simulink model "APSA"  (R2014b)
settings: Solver=FixedStepDiscrete  StartTime=0.0  StopTime=180  FixedStep=0.01  RelTol=1e-3
PreLoadFcn:
  | if exist('tl_preloadfcn','file'), tl_preloadfcn(gcs,400); end
PostLoadFcn:
  | if exist('tl_postloadfcn','file'), tl_postloadfcn(gcs,400); end
InitFcn:
  | if exist('tlds_init','file'), tlds_init(gcs); end
StartFcn:
  | if exist('tlds_start','file'), tlds_start(gcs); end
StopFcn:
  | if exist('tlds_stop','file'), tlds_stop(gcs); end
values from neighbouring files (symbols this model uses):
  EERAM_Map_Backward_Values = EERAM_Current_Map_Backward.signals.values(row,:)    [Create_Map.m]    (also in EERAM_Map_Backward_Values_2.mat = [0 0 0 0 0 0 150 150 150 150 150 150 ... (100 elements, 1x10)
  EERAM_Map_Forward_Values = EERAM_Current_Map_Forward.signals.values(row,:)    [Create_Map.m]    (also in EERAM_Map_Forward_Values_2.mat = [150 150 150 150 150 150 150 150 150 150 150 150 ... (100 el)
undefined symbols (not defined in the file or in its folder): sigbuilder_block
libraries: tllib x2
(part 1 of 3)
PreSaveFcn:
  | if exist('tl_presavefcn','file'), tl_presavefcn(gcs); end
settings Model: TL_MAIN_DATA={'codeopt',{'linebreaklimit',150,'cleancode',1},'logopt',{'globalloggingmode',4},'date',736348.7418854282,'advcodeopt',{'EnableExternCStateflowSymbols';'on'}}  TLRevision=400  DS_PROJECTFILE=APSA.dd  BufferReuse=off  Creator=VMware  LastModifiedBy=mdenichilo
settings DataIOCC: LimitDataPoints=off
settings OptimizationCC: BlockReduction=off  OptimizeBlockIOStorage=off  BufferReuse=off  GlobalBufferReuse=off  ExpressionFolding=off  LocalBlockOutputs=off
settings DebuggingCC: BusObjectLabelMismatch=error  StrictBusMsg=ErrorOnBusTreatedAsVector  NonBusSignalsTreatedAsBus=error
settings SFSimCC: SimCustomHeaderCode="#include \"APSA_Config.h\""

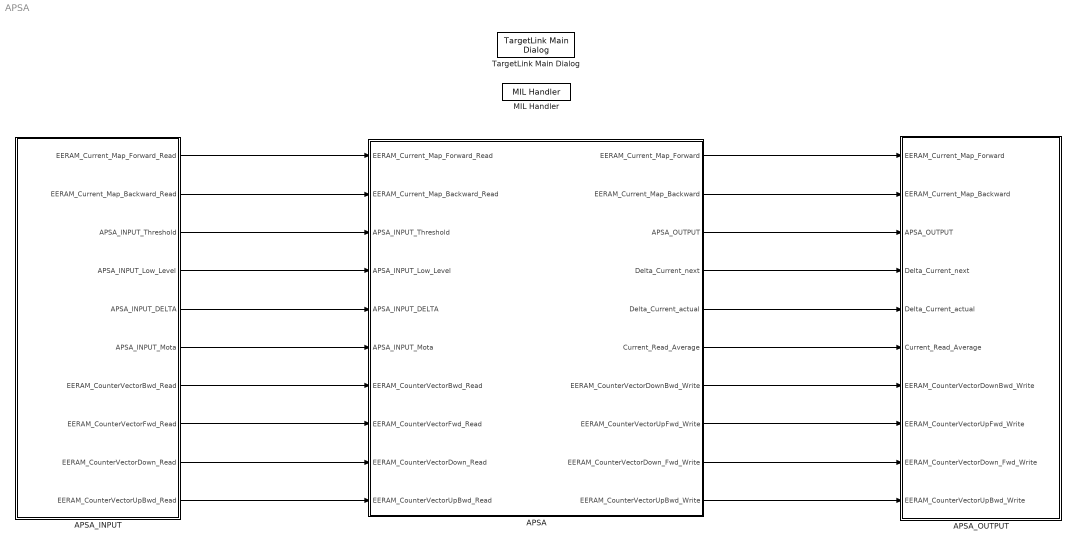
== system APSA ==
  APSA : Subsystem  Tag=TargetLink Simulation Frame  mask(TL_SimFrame){}
      settings: CopyFcn=if exist('tl_copyfcn','file'), tl_copyfcn(gcbh); end  NameChangeFcn=if exist('tl_framenamechangefcn','file'), tl_framenamechangefcn(gcbh); end
      settings: OpenFcn=|
      | if exist('open_tlsubsystem','file')
      |    open_tlsubsystem(gcbh);
      | else
      |    tlsubsystem = ...
      |       find_system(gcb, ...
      |       'LookUnderMasks','on', ...
      |       'FollowLinks','on', ...
      |       'Tag','MIL Subsystem');
      |    open_system(tlsubsystem);
      | end
      mask Display: disp('TargetLink\nModel-\nin-the-loop\nmode')
  APSA_INPUT : Subsystem
  APSA_OUTPUT : Subsystem
  MIL Handler : tllib/MIL Handler  data={'date',730486}
  TargetLink Main Dialog : tllib/TargetLink Main Dialog  data=[]
  wires:
  APSA_INPUT/2(EERAM_Current_Map_Backward_Read) -> APSA/2(EERAM_Current_Map_Backward_Read)
  APSA_INPUT/3(APSA_INPUT_Threshold) -> APSA/3(APSA_INPUT_Threshold)
  APSA_INPUT/6(APSA_INPUT_Mota) -> APSA/6(APSA_INPUT_Mota)
  APSA_INPUT/4(APSA_INPUT_Low_Level) -> APSA/4(APSA_INPUT_Low_Level)
  APSA_INPUT/5(APSA_INPUT_DELTA) -> APSA/5(APSA_INPUT_DELTA)
  APSA_INPUT/1(EERAM_Current_Map_Forward_Read) -> APSA/1(EERAM_Current_Map_Forward_Read)
  APSA/1(EERAM_Current_Map_Forward) -> APSA_OUTPUT/1(EERAM_Current_Map_Forward)
  APSA/2(EERAM_Current_Map_Backward) -> APSA_OUTPUT/2(EERAM_Current_Map_Backward)
  APSA/3(APSA_OUTPUT) -> APSA_OUTPUT/3(APSA_OUTPUT)
  APSA/6(Current_Read_Average) -> APSA_OUTPUT/6(Current_Read_Average)
  APSA/5(Delta_Current_actual) -> APSA_OUTPUT/5(Delta_Current_actual)
  APSA/4(Delta_Current_next) -> APSA_OUTPUT/4(Delta_Current_next)
  APSA/7(EERAM_CounterVectorDownBwd_Write) -> APSA_OUTPUT/7(EERAM_CounterVectorDownBwd_Write)
  APSA/8(EERAM_CounterVectorUpFwd_Write) -> APSA_OUTPUT/8(EERAM_CounterVectorUpFwd_Write)
  APSA/10(EERAM_CounterVectorUpBwd_Write) -> APSA_OUTPUT/10(EERAM_CounterVectorUpBwd_Write)
  APSA/9(EERAM_CounterVectorDown_Fwd_Write) -> APSA_OUTPUT/9(EERAM_CounterVectorDown_Fwd_Write)
  APSA_INPUT/8(EERAM_CounterVectorFwd_Read) -> APSA/8(EERAM_CounterVectorFwd_Read)
  APSA_INPUT/10(EERAM_CounterVectorUpBwd_Read) -> APSA/10(EERAM_CounterVectorUpBwd_Read)
  APSA_INPUT/7(EERAM_CounterVectorBwd_Read) -> APSA/7(EERAM_CounterVectorBwd_Read)
  APSA_INPUT/9(EERAM_CounterVectorDown_Read) -> APSA/9(EERAM_CounterVectorDown_Read)

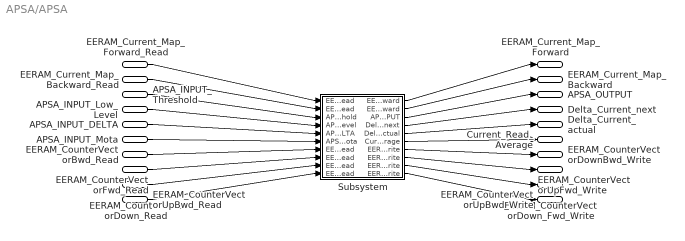
== system APSA/APSA ==
  EERAM_Current_Map_Forward_Read : Inport
  EERAM_Current_Map_Backward_Read : Inport  Port=2
  APSA_INPUT_Threshold : Inport  Port=3
  APSA_INPUT_Low_Level : Inport  Port=4
  APSA_INPUT_DELTA : Inport  Port=5
  APSA_INPUT_Mota : Inport  Port=6
  EERAM_CounterVectorBwd_Read : Inport  Port=7
  EERAM_CounterVectorFwd_Read : Inport  Port=8
  EERAM_CounterVectorDown_Read : Inport  Port=9
  EERAM_CounterVectorUpBwd_Read : Inport  Port=10
  Subsystem : Subsystem  mask(TL_Enable){}
      settings: OpenFcn=warndlg(get_param(gcb,'MaskHelp'),'Serious Warning');
      mask Help: This subsystem keeps the TargetLink subsystem (subsystem with TargetLink blocks for production code generation), and is needed for the TargetLink simulation frame to work properly. DO NOT DELETE OR MODIFY IT!
  EERAM_Current_Map_Forward : Outport
  EERAM_Current_Map_Backward : Outport  Port=2
  APSA_OUTPUT : Outport  Port=3
  Delta_Current_next : Outport  Port=4
  Delta_Current_actual : Outport  Port=5
  Current_Read_Average : Outport  Port=6
  EERAM_CounterVectorDownBwd_Write : Outport  Port=7
  EERAM_CounterVectorUpFwd_Write : Outport  Port=8
  EERAM_CounterVectorDown_Fwd_Write : Outport  Port=9
  EERAM_CounterVectorUpBwd_Write : Outport  Port=10
  wires:
  EERAM_Current_Map_Forward_Read/1 -> Subsystem/1(EERAM_Current_Map_Forward_Read)
  EERAM_Current_Map_Backward_Read/1 -> Subsystem/2(EERAM_Current_Map_Backward_Read)
  APSA_INPUT_Threshold/1 -> Subsystem/3(APSA_INPUT_Threshold)
  APSA_INPUT_Low_Level/1 -> Subsystem/4(APSA_INPUT_Low_Level)
  APSA_INPUT_DELTA/1 -> Subsystem/5(APSA_INPUT_DELTA)
  APSA_INPUT_Mota/1 -> Subsystem/6(APSA_INPUT_Mota)
  EERAM_CounterVectorBwd_Read/1 -> Subsystem/7(EERAM_CounterVectorBwd_Read)
  EERAM_CounterVectorFwd_Read/1 -> Subsystem/8(EERAM_CounterVectorFwd_Read)
  EERAM_CounterVectorDown_Read/1 -> Subsystem/9(EERAM_CounterVectorDown_Read)
  EERAM_CounterVectorUpBwd_Read/1 -> Subsystem/10(EERAM_CounterVectorUpBwd_Read)
  Subsystem/1(EERAM_Current_Map_Forward) -> EERAM_Current_Map_Forward/1
  Subsystem/2(EERAM_Current_Map_Backward) -> EERAM_Current_Map_Backward/1
  Subsystem/3(APSA_OUTPUT) -> APSA_OUTPUT/1
  Subsystem/4(Delta_Current_next) -> Delta_Current_next/1
  Subsystem/5(Delta_Current_actual) -> Delta_Current_actual/1
  Subsystem/6(Current_Read_Average) -> Current_Read_Average/1
  Subsystem/7(EERAM_CounterVectorDownBwd_Write) -> EERAM_CounterVectorDownBwd_Write/1
  Subsystem/8(EERAM_CounterVectorUpFwd_Write) -> EERAM_CounterVectorUpFwd_Write/1
  Subsystem/9(EERAM_CounterVectorDown_Fwd_Write) -> EERAM_CounterVectorDown_Fwd_Write/1
  Subsystem/10(EERAM_CounterVectorUpBwd_Write) -> EERAM_CounterVectorUpBwd_Write/1

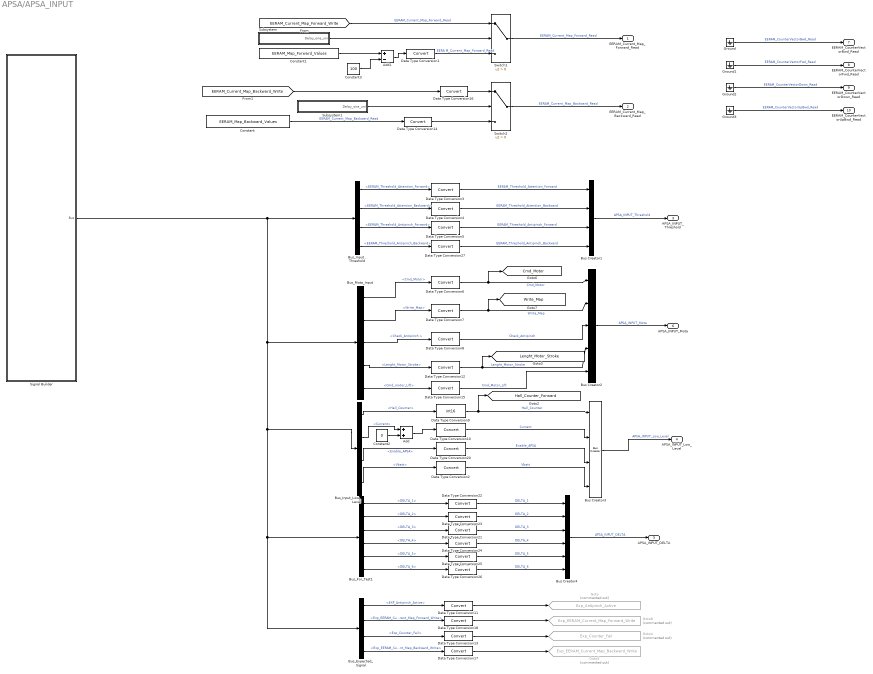
== system APSA/APSA_INPUT ==
  Add : Sum
  Add1 : Sum  Inputs=+-
  Bus Creator1 : BusCreator
  Bus Creator2 : BusCreator  Inputs=5
  Bus Creator3 : BusCreator
  Bus Creator4 : BusCreator  Inputs=6
  Bus_Expected_Signal : BusSelector  OutputSignals=EXP_Antipinch_Active,Exp_EERAM_Current_Map_Forward_Write,Exp_Counter_Fail,Exp_EERAM_Current_Map_Backward_Write
  Bus_For_Test1 : BusSelector  OutputSignals=DELTA_1,DELTA_2,DELTA_3,DELTA_4,DELTA_5,DELTA_6
  Bus_Input_Low_Level : BusSelector  OutputSignals=Hall_Counter,Current,Enable_APSA,Vbatt
  Bus_Input_Threshold : BusSelector  OutputSignals=EERAM_Threshold_Attention_Forward,EERAM_Threshold_Attention_Backward,EERAM_Threshold_Antipinch_Forward,EERAM_Threshold_Antipinch_Backward
  Bus_Mota_Input : BusSelector  OutputSignals=Cmd_Motor,Write_Map,Check_Antipinch ,Lenght_Motor_Stroke,Cmd_motor_Lift
  Constant : Constant  Value=EERAM_Map_Backward_Values  OutDataTypeStr=double
  Constant1 : Constant  Value=EERAM_Map_Forward_Values  OutDataTypeStr=double
  Constant2 : Constant  Value=0
  Constant3 : Constant  Value=100
  Data Type Conversion{1..8,10..18,20..27} (25 alike) : DataTypeConversion
  Data Type Conversion9 : DataTypeConversion  OutDataTypeStr=int16
  Goto : Goto  Commented=on  GotoTag=Exp_Antipinch_Active  TagVisibility=global
  Goto4 : Goto  Commented=on  GotoTag=Exp_Counter_Fail  TagVisibility=global
  Goto5 : Goto  Commented=on  GotoTag=Exp_EERAM_Current_Map_Backward_Write  TagVisibility=global
  Goto8 : Goto  Commented=on  GotoTag=Exp_EERAM_Current_Map_Forward_Write  TagVisibility=global
  Ground{,1..3} (4 alike) : Ground
  Signal Builder : Subsystem  Tag=STV Subsys  LoadFcn=sigbuilder_block('load');  StartFcn=sigbuilder_block('start');  StopFcn=sigbuilder_block('stop');  ClipboardFcn=sigbuilder_block('clipboard');  mask(Sigbuilder block){}
      mask help: Simulink:masks:SigbuilderBlock_MD
      mask init:
      | if ~strcmp(get_param(bdroot(gcbh),'SimulationStatus'),'stopped') tuvar = sigbuilder_block('maskInit'); end
      settings: CopyFcn=sigbuilder_block('copy');  DeleteFcn=sigbuilder_block('delete');  ModelCloseFcn=sigbuilder_block('modelClose');  PreSaveFcn=sigbuilder_block('preSave');  PauseFcn=sigbuilder_block('pause');  ContinueFcn=sigbuilder_block('continue');  NameChangeFcn=sigbuilder_block('namechange');  OpenFcn=sigbuilder_block('open',[437.6 199.2 550.4 400 ]);  CloseFcn=sigbuilder_block('close');
      mask Display: plot(0, 0, 100, 100,[2, 2, 32, 32, 2], [68, 8, 8, 68, 68],[32, 2], [38, 38], [32, 19, 2],[53, 60, 44], [32, 17, 17, 2],[16, 16, 31, 31]);txt = getActiveGroup(gcbh);text(2, 100, txt,'verticalAlignment', 'top');
  Subsystem : Subsystem
  Subsystem1 : Subsystem
  Switch1 : Switch  Criteria=u2 > Threshold
  Switch2 : Switch  Criteria=u2 > Threshold
  EERAM_Current_Map_Forward_Read : Outport
  EERAM_Current_Map_Backward_Read : Outport  Port=2
  APSA_INPUT_Threshold : Outport  Port=3
  APSA_INPUT_Low_Level : Outport  Port=4
  APSA_INPUT_DELTA : Outport  Port=5
  APSA_INPUT_Mota : Outport  Port=6
  EERAM_CounterVectorBwd_Read : Outport  Port=7
  EERAM_CounterVectorFwd_Read : Outport  Port=8
  EERAM_CounterVectorDown_Read : Outport  Port=9
  EERAM_CounterVectorUpBwd_Read : Outport  Port=10
  tag scope: Cmd_Motor=global, Hall_Counter_Forward=global, Lenght_Motor_Stroke=global, Write_Map=global
  wires:
  Bus_Input_Threshold/1 -> Data Type Conversion3/1  "<EERAM_Threshold_Attention_Forward>"
  Bus_Input_Threshold/3 -> Data Type Conversion5/1  "<EERAM_Threshold_Antipinch_Forward>"
  Bus_Mota_Input/1 -> Data Type Conversion6/1  "<Cmd_Motor>"
  Bus_Mota_Input/2 -> Data Type Conversion7/1  "<Write_Map>"
  Bus_Mota_Input/3 -> Data Type Conversion8/1  "<Check_Antipinch >"
  Data Type Conversion3/1 -> Bus Creator1/1  "EERAM_Threshold_Attention_Forward"
  Data Type Conversion5/1 -> Bus Creator1/3  "EERAM_Threshold_Antipinch_Forward"
  Data Type Conversion7/1 -> [Write_Map], Bus Creator2/2  "Write_Map"
  Data Type Conversion8/1 -> Bus Creator2/3  "Check_Antipinch"
  Data Type Conversion6/1 -> [Cmd_Motor], Bus Creator2/1  "Cmd_Motor"
  Bus Creator1/1 -> APSA_INPUT_Threshold/1  "APSA_INPUT_Threshold"
  Bus Creator2/1 -> APSA_INPUT_Mota/1  "APSA_INPUT_Mota"
  Bus_Input_Low_Level/1 -> Data Type Conversion9/1  "<Hall_Counter>"
  Bus_Input_Low_Level/2 -> Add/1  "<Current>"
  Data Type Conversion10/1 -> Bus Creator3/2  "Current"
  Data Type Conversion9/1 -> [Hall_Counter_Forward], Bus Creator3/1  "Hall_Counter"
  Bus_Mota_Input/4 -> Data Type Conversion12/1  "<Lenght_Motor_Stroke>"
  Data Type Conversion12/1 -> [Lenght_Motor_Stroke], Bus Creator2/4  "Lenght_Motor_Stroke"
  Bus Creator3/1 -> APSA_INPUT_Low_Level/1  "APSA_INPUT_Low_Level"
  Bus_Expected_Signal/1 -> Data Type Conversion11/1  "<EXP_Antipinch_Active>"
  Data Type Conversion11/1 -> Goto/1
  Bus_Expected_Signal/2 -> Data Type Conversion18/1  "<Exp_EERAM_Current_Map_Forward_Write>"
  Bus_Input_Threshold/2 -> Data Type Conversion4/1  "<EERAM_Threshold_Attention_Backward>"
  Data Type Conversion4/1 -> Bus Creator1/2  "EERAM_Threshold_Attention_Backward"
  Bus_Expected_Signal/3 -> Data Type Conversion13/1  "<Exp_Counter_Fail>"
  Data Type Conversion13/1 -> Goto4/1
  Data Type Conversion1/1 -> Switch1/3  "EERA M_Current_Map_Forward_Read"
  Subsystem/1(Delay_one_unit) -> Switch1/2
  [EERAM_Current_Map_Forward_Write] -> Switch1/1  "EERAM_Current_Map_Forward_Read"
  Signal Builder/1(Bus) -> Bus_Input_Threshold/1, Bus_Input_Low_Level/1, Bus_For_Test1/1, Bus_Expected_Signal/1, Bus_Mota_Input/1
  Subsystem1/1(Delay_one_unit) -> Switch2/2
  [EERAM_Current_Map_Backward_Write] -> Data Type Conversion16/1
  Data Type Conversion16/1 -> Switch2/1
  Bus_Expected_Signal/4 -> Data Type Conversion17/1  "<Exp_EERAM_Current_Map_Backward_Write>"
  Data Type Conversion17/1 -> Goto5/1
  Bus_Input_Low_Level/3 -> Data Type Conversion20/1  "<Enable_APSA>"
  Data Type Conversion20/1 -> Bus Creator3/3  "Enable_APSA"
  Bus_For_Test1/1 -> Data Type Conversion22/1  "<DELTA_1>"
  Bus_For_Test1/2 -> Data Type Conversion23/1  "<DELTA_2>"
  Bus_For_Test1/3 -> Data Type Conversion21/1  "<DELTA_3>"
  Bus_For_Test1/4 -> Data Type Conversion24/1  "<DELTA_4>"
  Bus_For_Test1/5 -> Data Type Conversion25/1  "<DELTA_5>"
  Bus_For_Test1/6 -> Data Type Conversion26/1  "<DELTA_6>"
  Data Type Conversion23/1 -> Bus Creator4/2  "DELTA_2"
  Data Type Conversion26/1 -> Bus Creator4/6  "DELTA_6"
  Data Type Conversion22/1 -> Bus Creator4/1  "DELTA_1"
  Data Type Conversion24/1 -> Bus Creator4/4  "DELTA_4"
  Data Type Conversion25/1 -> Bus Creator4/5  "DELTA_5"
  Data Type Conversion21/1 -> Bus Creator4/3  "DELTA_3"
  Bus Creator4/1 -> APSA_INPUT_DELTA/1  "APSA_INPUT_DELTA"
  Constant1/1 -> Add1/1
  Bus_Input_Threshold/4 -> Data Type Conversion27/1  "<EERAM_Threshold_Antipinch_Backward>"
  Data Type Conversion27/1 -> Bus Creator1/4  "EERAM_Threshold_Antipinch_Backward"
  Constant/1 -> Data Type Conversion14/1  "EERAM_Current_Map_Backward_Read"
  Data Type Conversion18/1 -> Goto8/1
  Switch1/1 -> EERAM_Current_Map_Forward_Read/1  "EERAM_Current_Map_Forward_Read"
  Switch2/1 -> EERAM_Current_Map_Backward_Read/1  "EERAM_Current_Map_Backward_Read"
  Constant2/1 -> Add/2
  Add/1 -> Data Type Conversion10/1
  Constant3/1 -> Add1/2
  Data Type Conversion14/1 -> Switch2/3
  Add1/1 -> Data Type Conversion1/1
  Ground/1 -> EERAM_CounterVectorBwd_Read/1  "EERAM_CounterVectorBwd_Read"
  Ground1/1 -> EERAM_CounterVectorFwd_Read/1  "EERAM_CounterVectorFwd_Read"
  Ground2/1 -> EERAM_CounterVectorDown_Read/1  "EERAM_CounterVectorDown_Read"
  Ground3/1 -> EERAM_CounterVectorUpBwd_Read/1  "EERAM_CounterVectorUpBwd_Read"
  Bus_Input_Low_Level/4 -> Data Type Conversion2/1  "<Vbatt>"
  Data Type Conversion2/1 -> Bus Creator3/4  "Vbatt"
  Bus_Mota_Input/5 -> Data Type Conversion15/1  "<Cmd_motor_Lift>"
  Data Type Conversion15/1 -> Bus Creator2/5  "Cmd_Motor_Lift"

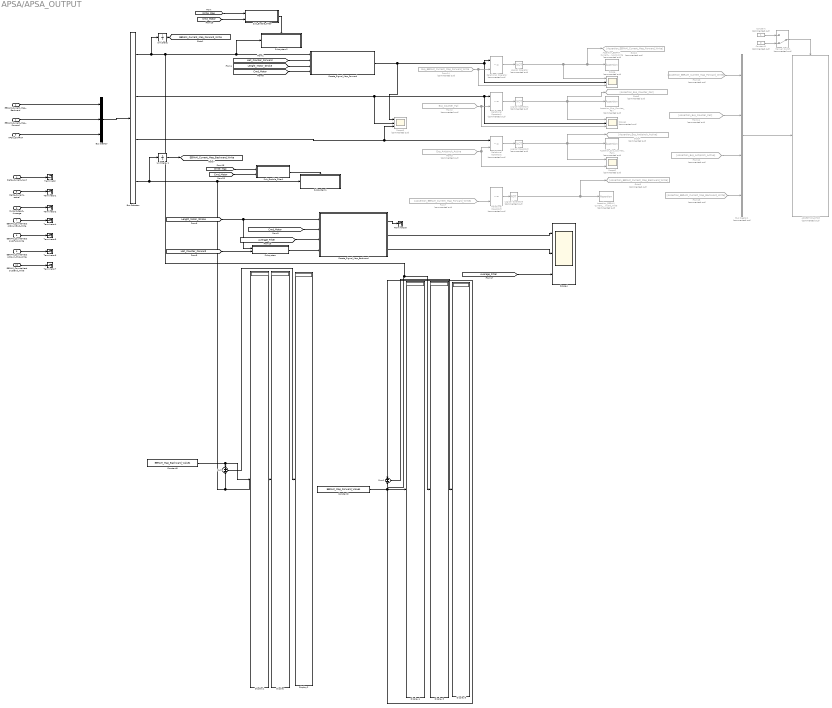
== system APSA/APSA_OUTPUT ==
  EERAM_Current_Map_Forward : Inport
  EERAM_Current_Map_Backward : Inport  Port=2
  APSA_OUTPUT : Inport  Port=3
  Delta_Current_next : Inport  Port=4
  Delta_Current_actual : Inport  Port=5
  Current_Read_Average : Inport  Port=6
  EERAM_CounterVectorDownBwd_Write : Inport  Port=7
  EERAM_CounterVectorUpFwd_Write : Inport  Port=8
  EERAM_CounterVectorDown_Fwd_Write : Inport  Port=9
  EERAM_CounterVectorUpBwd_Write : Inport  Port=10
  ASSERTION_STOP : Subsystem  Commented=on
  Assertion_EERAM_Current_Map_Backward_Write : Assertion  Commented=on  StopWhenAssertionFail=off
  Assertion_EERAM_Current_Map_Forward_Write : Assertion  Commented=on  StopWhenAssertionFail=off
  Assertion_Exp_Counter_Fail : Assertion  Commented=on  StopWhenAssertionFail=off
  Assertion_Exp_Counter_Fail1 : Assertion  Commented=on  StopWhenAssertionFail=off
  Bus Creator : BusCreator  Inputs=3
  Bus Creator1 : BusCreator  Commented=on
  Bus Selector : BusSelector  OutputSignals=EERAM_Current_Map_Forward_Write,APSA_OUTPUT.Fail_Sens_Current,APSA_OUTPUT.Antipinch_Active,EERAM_Current_Map_Backward_Write
  Constant : Constant  Commented=on
  Constant1 : Constant  Commented=on  Value=0
  Constant2 : Constant  Value=EERAM_Map_Forward_Values  OutDataTypeStr=double
  Constant3 : Constant  Value=EERAM_Map_Backward_Values  OutDataTypeStr=double
  Create_Signal_Map_Backward : Stateflow chart  TreatAsAtomicUnit=on
  Create_Signal_Map_Forward : Stateflow chart  TreatAsAtomicUnit=on
  Display{,1..5} (6 alike) : Display
  From10 : From  Commented=on  GotoTag=Assertion_EERAM_Current_Map_Forward_Write
  From11 : From  Commented=on  GotoTag=Assertion_Exp_Counter_Fail
  From12 : From  Commented=on  GotoTag=Assertion_Exp_Antipinch_Active
  From13 : From  Commented=on  GotoTag=Assertion_EERAM_Current_Map_Backward_Write
  From14 : From  Commented=on  GotoTag=Exp_EERAM_Current_Map_Forward_Write
  From2 : From  Commented=on  GotoTag=Exp_Counter_Fail  TagVisibility=global
  From3 : From  Commented=on  GotoTag=Exp_Antipinch_Active  TagVisibility=global
  From7 : From  Commented=on  GotoTag=Assertion_EERAM_Current_Map_Forward_Write
  Goto2 : Goto  Commented=on  GotoTag=Assertion_EERAM_Current_Map_Forward_Write
  Goto3 : Goto  Commented=on  GotoTag=Assertion_Exp_Counter_Fail
  Goto4 : Goto  Commented=on  GotoTag=Assertion_Exp_Antipinch_Active
  Goto5 : Goto  Commented=on  GotoTag=Assertion_EERAM_Current_Map_Backward_Write
  Logical Operator{,1..3} (4 alike) : Logic  Commented=on  Operator=NOT  AllPortsSameDT=off  OutDataTypeStr=boolean
  Manual Switch : ManualSwitch  Commented=on  CurrentSetting=0
  Relational Operator{,1..3} (4 alike) : RelationalOperator  Commented=on  Operator=~=  OutDataTypeStr=boolean
  Scope{,1..3} (4 alike) : Scope  Commented=on  NumInputPorts=3
      Scope settings: TimeRange=0.008849178119752832  YMin=-1~0~5.6  YMax=1~5~5.74  SampleInput=on
      Scope1 settings: YMin=-5~-5~-5  YMax=5~5~5
      Scope2 settings: YMin=-5~-5~-5  YMax=5~5~5  SaveName=ScopeData2
      Scope3 settings: YMin=-5~-5~-5  YMax=5~5~5  SaveName=ScopeData3
  Scope4 : Scope  NumInputPorts=3
      settings: TimeRange=0.1993998881147334  YMin=-1~-1~43  YMax=1~1~47  SaveName=ScopeData5  SampleInput=on
  Sub_Enable_Filter : Subsystem
  Sub_Enable_Filter1 : Subsystem
  Subsystem : Subsystem
  Subsystem1 : Subsystem
  Subsystem2 : Subsystem
  Sum : Sum  Inputs=+-
  Sum1 : Sum  Inputs=+-
  Terminator{,1..7} (8 alike) : Terminator
  Unit Delay : UnitDelay  SampleTime=-1
  Unit Delay1 : UnitDelay  SampleTime=-1
  tag scope: EERAM_Current_Map_Backward_Write=global, EERAM_Current_Map_Forward_Write=global
  wires:
  Logical Operator/1 -> Goto2/1, Assertion_EERAM_Current_Map_Forward_Write/1, Scope/1  "Assertion_EERAM_Current_Map_Forward_Write"
  Relational Operator/1 -> Logical Operator/1
  Create_Signal_Map_Forward/1(Map_Signal) -> Scope3/1, Relational Operator/1, Scope/2
  [Hall_Counter_Forward] -> Create_Signal_Map_Forward/2(Hall_Counter)
  [Lenght_Motor_Stroke] -> Create_Signal_Map_Forward/3(Lenght_Motor_Stroke)
  APSA_OUTPUT/1 -> Bus Creator/3
  Bus Selector/2 -> Scope3/2, Scope1/2, Relational Operator1/1  "<Fail_Sens_Current>"
  From2/1 -> Scope1/3, Relational Operator1/2  "Exp_Counter_Fail"
  Relational Operator1/1 -> Logical Operator1/1
  Logical Operator1/1 -> Scope1/1, Goto3/1, Assertion_Exp_Counter_Fail/1  "Assertion_Exp_Counter_Fail"
  From3/1 -> Scope2/3, Relational Operator2/2  "Exp_Antipinch_Active"
  Relational Operator2/1 -> Logical Operator2/1
  Logical Operator2/1 -> Goto4/1, Scope2/1, Assertion_Exp_Counter_Fail1/1  "Assertion_Exp_Antipinch_Active"
  Bus Selector/4 -> Unit Delay1/1, Display/1, Sum/2, Subsystem1/1(In1)  "<EERAM_Current_Map_Backward_Write>"
  Subsystem/1(Hall_Counter_Backward) -> Create_Signal_Map_Backward/4(Hall_Counter_Backward)
  Logical Operator3/1 -> Goto5/1, Assertion_EERAM_Current_Map_Backward_Write/1  "Assertion_EERAM_Current_Map_Backward_Write"
  Relational Operator3/1 -> Logical Operator3/1
  [Cmd_Motor] -> Create_Signal_Map_Forward/4(Cmd_Motor)
  [Cmd_Motor] -> Create_Signal_Map_Backward/2(Cmd_Motor)
  EERAM_Current_Map_Forward/1 -> Bus Creator/2
  EERAM_Current_Map_Backward/1 -> Bus Creator/1
  Bus Creator/1 -> Bus Selector/1
  [Hall_Counter_Forward] -> Subsystem/2(Hall_Counter)
  Bus Creator1/1 -> ASSERTION_STOP/1(Assertion_Stop)
  From10/1 -> Bus Creator1/1
  From11/1 -> Bus Creator1/2
  From12/1 -> Bus Creator1/3
  From13/1 -> Bus Creator1/4
  Manual Switch/1 -> ASSERTION_STOP/Enable
  Constant/1 -> Manual Switch/1
  Constant1/1 -> Manual Switch/2
  Bus Selector/3 -> Scope3/3, Relational Operator2/1  "<Antipinch_Active>"
  From14/1 -> Scope/3, Relational Operator/2
  From7/1 -> Relational Operator3/2
  [Average_Filter] -> Create_Signal_Map_Backward/3(Current)
  Create_Signal_Map_Backward/2(Index_vector) -> Scope4/1  "indexvector"
  [Average_Filter] -> Scope4/3
  [Lenght_Motor_Stroke] -> Subsystem/1(Lenght_Motor_Stroke), Create_Signal_Map_Backward/1(Lenght_Motor_Stroke)
  Create_Signal_Map_Backward/3(Mappa) -> Scope4/2  "mappa_attuale"
  Sub_Enable_Filter1/1(Enable_Filter) -> Subsystem1/Enable
  Bus Selector/1 -> Unit Delay/1, Sum1/2, Display3/1, Subsystem2/1(In1), Create_Signal_Map_Forward/1(EERAM_Current_Map_Forward_Write)  "<EERAM_Current_Map_Forward_Write>"
  [Write_Map] -> Sub_Enable_Filter/1(Write_Map)
  [Cmd_Motor] -> Sub_Enable_Filter/2(Cmd_Motor)
  Sub_Enable_Filter/1(Enable_Filter) -> Subsystem2/Enable
  [Write_Map] -> Sub_Enable_Filter1/1(Write_Map)
  [Cmd_Motor] -> Sub_Enable_Filter1/2(Cmd_Motor)
  Constant3/1 -> Display1/1, Sum/1
  Delta_Current_next/1 -> Terminator/1
  Delta_Current_actual/1 -> Terminator1/1
  Current_Read_Average/1 -> Terminator2/1
  Sum/1 -> Display2/1
  Constant2/1 -> Sum1/1, Display4/1
  Sum1/1 -> Display5/1
  Create_Signal_Map_Backward/1(EERAM_Current_Map_Backward_Write) -> Terminator3/1
  Unit Delay/1 -> [EERAM_Current_Map_Forward_Write]
  Unit Delay1/1 -> [EERAM_Current_Map_Backward_Write]
  EERAM_CounterVectorDownBwd_Write/1 -> Terminator4/1
  EERAM_CounterVectorUpFwd_Write/1 -> Terminator5/1
  EERAM_CounterVectorDown_Fwd_Write/1 -> Terminator6/1
  EERAM_CounterVectorUpBwd_Write/1 -> Terminator7/1

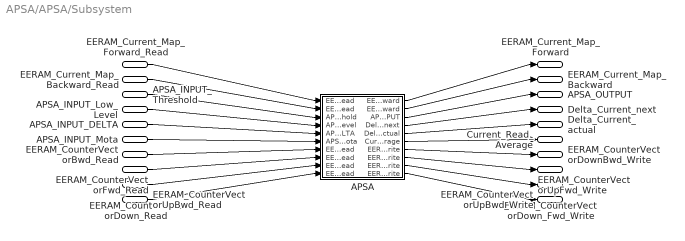
== system APSA/APSA/Subsystem ==
  EERAM_Current_Map_Forward_Read : Inport
  EERAM_Current_Map_Backward_Read : Inport  Port=2
  APSA_INPUT_Threshold : Inport  Port=3
  APSA_INPUT_Low_Level : Inport  Port=4
  APSA_INPUT_DELTA : Inport  Port=5
  APSA_INPUT_Mota : Inport  Port=6
  EERAM_CounterVectorBwd_Read : Inport  Port=7
  EERAM_CounterVectorFwd_Read : Inport  Port=8
  EERAM_CounterVectorDown_Read : Inport  Port=9
  EERAM_CounterVectorUpBwd_Read : Inport  Port=10
  APSA : Subsystem  Tag=MIL Subsystem  Description=a  mask(MIL Subsystem){}
      settings: CopyFcn=if exist('tl_copyfcn','file'), tl_copyfcn(gcbh); end  NameChangeFcn=if exist('tl_namechangefcn','file'), tl_namechangefcn(gcbh); end  DestroyFcn=if exist('update_tl_main_dlg','file'), update_tl_main_dlg('TL_subs_display'); end
      mask Display: disp('TargetLink Subsystem')
  EERAM_Current_Map_Forward : Outport
  EERAM_Current_Map_Backward : Outport  Port=2
  APSA_OUTPUT : Outport  Port=3
  Delta_Current_next : Outport  Port=4
  Delta_Current_actual : Outport  Port=5
  Current_Read_Average : Outport  Port=6
  EERAM_CounterVectorDownBwd_Write : Outport  Port=7
  EERAM_CounterVectorUpFwd_Write : Outport  Port=8
  EERAM_CounterVectorDown_Fwd_Write : Outport  Port=9
  EERAM_CounterVectorUpBwd_Write : Outport  Port=10
  wires:
  EERAM_Current_Map_Forward_Read/1 -> APSA/1(EERAM_Current_Map_Forward_Read)
  EERAM_Current_Map_Backward_Read/1 -> APSA/2(EERAM_Current_Map_Backward_Read)
  APSA_INPUT_Threshold/1 -> APSA/3(APSA_INPUT_Threshold)
  APSA_INPUT_Low_Level/1 -> APSA/4(APSA_INPUT_Low_Level)
  APSA_INPUT_DELTA/1 -> APSA/5(APSA_INPUT_DELTA)
  APSA_INPUT_Mota/1 -> APSA/6(APSA_INPUT_Mota)
  EERAM_CounterVectorBwd_Read/1 -> APSA/7(EERAM_CounterVectorBwd_Read)
  EERAM_CounterVectorFwd_Read/1 -> APSA/8(EERAM_CounterVectorFwd_Read)
  EERAM_CounterVectorDown_Read/1 -> APSA/9(EERAM_CounterVectorDown_Read)
  EERAM_CounterVectorUpBwd_Read/1 -> APSA/10(EERAM_CounterVectorUpBwd_Read)
  APSA/1(EERAM_Current_Map_Forward) -> EERAM_Current_Map_Forward/1
  APSA/2(EERAM_Current_Map_Backward) -> EERAM_Current_Map_Backward/1
  APSA/3(APSA_OUTPUT) -> APSA_OUTPUT/1
  APSA/4(Delta_Current_next) -> Delta_Current_next/1
  APSA/5(Delta_Current_actual) -> Delta_Current_actual/1
  APSA/6(Current_Read_Average) -> Current_Read_Average/1
  APSA/7(EERAM_CounterVectorDownBwd_Write) -> EERAM_CounterVectorDownBwd_Write/1
  APSA/8(EERAM_CounterVectorUpFwd_Write) -> EERAM_CounterVectorUpFwd_Write/1
  APSA/9(EERAM_CounterVectorDown_Fwd_Write) -> EERAM_CounterVectorDown_Fwd_Write/1
  APSA/10(EERAM_CounterVectorUpBwd_Write) -> EERAM_CounterVectorUpBwd_Write/1

== system APSA/APSA_INPUT/Signal Builder ==
  Bus Creator : BusCreator  Tag=Bus Creator  Inputs=28
  FromWs : FromWorkspace  Tag=STV FromWs  VariableName=tuvar  SampleTime=0
  Subsystem : Subsystem
  Bus : Outport
  wires:
  FromWs/1 -> Subsystem/1(In1)
  Bus Creator/1 -> Bus/1
  Subsystem/1(Enable_APSA) -> Bus Creator/1  "Enable_APSA"
  Subsystem/2(Cmd_Motor) -> Bus Creator/2  "Cmd_Motor"
  Subsystem/3(Hall_Counter) -> Bus Creator/3  "Hall_Counter"
  Subsystem/4("Check_Antipinch ") -> Bus Creator/4  "Check_Antipinch"
  Subsystem/5(Current) -> Bus Creator/5  "Current"
  Subsystem/6(Write_Map) -> Bus Creator/6  "Write_Map"
  Subsystem/7(Lenght_Motor_Stroke) -> Bus Creator/7  "Lenght_Motor_Stroke"
  Subsystem/8(EERAM_Threshold_Attention_Forward) -> Bus Creator/8  "EERAM_Threshold_Attention_Forward"
  Subsystem/9(EERAM_Threshold_Attention_Backward) -> Bus Creator/9  "EERAM_Threshold_Attention_Backward"
  Subsystem/10(EERAM_Threshold_Antipinch_Forward) -> Bus Creator/10  "EERAM_Threshold_Antipinch_Forward"
  Subsystem/11(EERAM_Threshold_Antipinch_Backward) -> Bus Creator/11  "EERAM_Threshold_Antipinch_Backward"
  Subsystem/12(DELTA_1) -> Bus Creator/12  "DELTA_1"
  Subsystem/13(DELTA_2) -> Bus Creator/13  "DELTA_2"
  Subsystem/14(DELTA_3) -> Bus Creator/14  "DELTA_3"
  Subsystem/15(Current1) -> Bus Creator/15  "Current1"
  Subsystem/16(DELTA_4) -> Bus Creator/16  "DELTA_4"
  Subsystem/17(DELTA_5) -> Bus Creator/17  "DELTA_5"
  Subsystem/18(DELTA_6) -> Bus Creator/18  "DELTA_6"
  Subsystem/19(EXP_Antipinch_Active) -> Bus Creator/19  "EXP_Antipinch_Active"
  Subsystem/20(Exp_EERAM_Current_Map_Forward_Write) -> Bus Creator/20  "Exp_EERAM_Current_Map_Forward_Write"
  Subsystem/21(Exp_EERAM_Current_Map_Backward_Write) -> Bus Creator/21  "Exp_EERAM_Current_Map_Backward_Write"
  Subsystem/22(Exp_Counter_Fail) -> Bus Creator/22  "Exp_Counter_Fail"
  Subsystem/23(mappa) -> Bus Creator/23  "mappa"
  Subsystem/24(3EEP_10V) -> Bus Creator/24  "3EEP_10V"
  Subsystem/25(3EEP_12V) -> Bus Creator/25  "3EEP_12V"
  Subsystem/26(3xEEP_16V) -> Bus Creator/26  "3xEEP_16V"
  Subsystem/27(Vbatt) -> Bus Creator/27  "Vbatt"
  Subsystem/28(Cmd_motor_Lift) -> Bus Creator/28  "Cmd_motor_Lift"

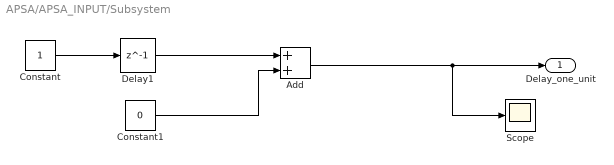
== system APSA/APSA_INPUT/Subsystem ==
  Add : Sum
  Constant : Constant
  Constant1 : Constant  Value=0
  Delay1 : Delay  DelayLength=1  InitialCondition=0
  Scope : Scope
      settings: YMin=0  YMax=1  SaveName=ScopeData4
  Delay_one_unit : Outport
  wires:
  Add/1 -> Scope/1, Delay_one_unit/1
  Constant/1 -> Delay1/1
  Constant1/1 -> Add/2
  Delay1/1 -> Add/1

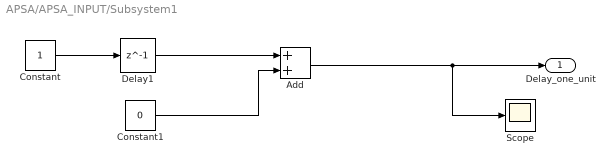
== system APSA/APSA_INPUT/Subsystem1 ==
  Add : Sum
  Constant : Constant
  Constant1 : Constant  Value=0
  Delay1 : Delay  DelayLength=1  InitialCondition=0
  Scope : Scope
      settings: SaveName=ScopeData4
  Delay_one_unit : Outport
  wires:
  Delay1/1 -> Add/1
  Constant1/1 -> Add/2
  Constant/1 -> Delay1/1
  Add/1 -> Delay_one_unit/1, Scope/1

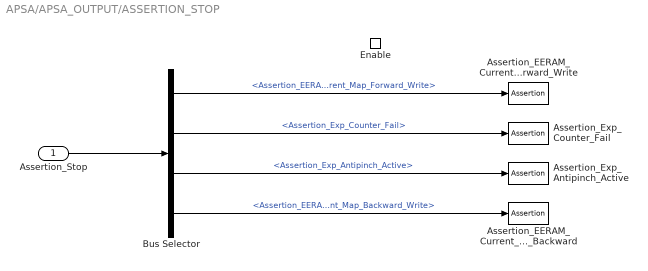
== system APSA/APSA_OUTPUT/ASSERTION_STOP ==
  Assertion_Stop : Inport
  Enable : EnablePort
  Assertion_EERAM_Current_Map_Backward : Assertion
  Assertion_EERAM_Current_Map_Forward_Write : Assertion
  Assertion_Exp_Antipinch_Active : Assertion
  Assertion_Exp_Counter_Fail : Assertion
  Bus Selector : BusSelector  OutputSignals=Assertion_EERAM_Current_Map_Forward_Write,Assertion_Exp_Counter_Fail,Assertion_Exp_Antipinch_Active,Assertion_EERAM_Current_Map_Backward_Write
  wires:
  Assertion_Stop/1 -> Bus Selector/1
  Bus Selector/1 -> Assertion_EERAM_Current_Map_Forward_Write/1  "<Assertion_EERAM_Current_Map_Forward_Write>"
  Bus Selector/2 -> Assertion_Exp_Counter_Fail/1  "<Assertion_Exp_Counter_Fail>"
  Bus Selector/3 -> Assertion_Exp_Antipinch_Active/1  "<Assertion_Exp_Antipinch_Active>"
  Bus Selector/4 -> Assertion_EERAM_Current_Map_Backward/1  "<Assertion_EERAM_Current_Map_Backward_Write>"

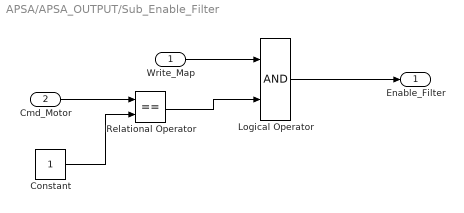
== system APSA/APSA_OUTPUT/Sub_Enable_Filter ==
  Write_Map : Inport
  Cmd_Motor : Inport  Port=2
  Constant : Constant
  Logical Operator : Logic  AllPortsSameDT=off  OutDataTypeStr=boolean
  Relational Operator : RelationalOperator  Operator===  OutDataTypeStr=boolean
  Enable_Filter : Outport
  wires:
  Cmd_Motor/1 -> Relational Operator/1
  Write_Map/1 -> Logical Operator/1
  Logical Operator/1 -> Enable_Filter/1
  Constant/1 -> Relational Operator/2
  Relational Operator/1 -> Logical Operator/2

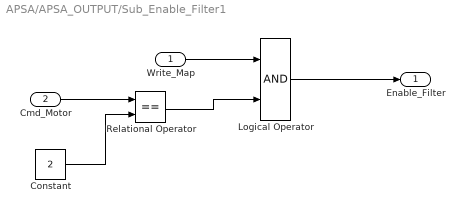
== system APSA/APSA_OUTPUT/Sub_Enable_Filter1 ==
  Write_Map : Inport
  Cmd_Motor : Inport  Port=2
  Constant : Constant  Value=2
  Logical Operator : Logic  AllPortsSameDT=off  OutDataTypeStr=boolean
  Relational Operator : RelationalOperator  Operator===  OutDataTypeStr=boolean
  Enable_Filter : Outport
  wires:
  Cmd_Motor/1 -> Relational Operator/1
  Write_Map/1 -> Logical Operator/1
  Logical Operator/1 -> Enable_Filter/1
  Constant/1 -> Relational Operator/2
  Relational Operator/1 -> Logical Operator/2

== system APSA/APSA_OUTPUT/Subsystem ==
  Lenght_Motor_Stroke : Inport
  Hall_Counter : Inport  Port=2
  Sum : Sum  Inputs=+-  OutDataTypeStr=int16  mask(TL_Sum){data={'date',736221.56170504633}}
      settings: CopyFcn=if exist('tl_reset_reviewflag') == 2, tl_reset_reviewflag(gcbh); end  DeleteFcn=if exist('delete_tlblock','file')==2,delete_tlblock(gcbh);end  NameChangeFcn=if exist('rename_tlblock','file')==2,rename_tlblock(gcbh);end  OpenFcn=if exist('tl_open_blockdlg','file')==2,tl_open_blockdlg(gcbh);else,open_system(gcbh,'parameter');end
      mask Help: eval(['if exist(''tl_online_help'',''file'') == 2, tl_online_help(''Topic'',''TL_Sum''),else, web([''jar:file:///'',matlabroot,''/help/toolbox/simulink/help.jar!/slref/' lower(get_param(gcbh,'Blocktype')) '.html''], ''-helpbrowser''),end'])
      mask Display: plot([-0.1, 1.05, NaN, -0.1, 1.05],[.01, .01, NaN, .99, .99]);
  Hall_Counter_Backward : Outport
  wires:
  Lenght_Motor_Stroke/1 -> Sum/1
  Hall_Counter/1 -> Sum/2
  Sum/1 -> Hall_Counter_Backward/1

== system APSA/APSA_OUTPUT/Subsystem1 ==
  In1 : Inport
  Enable : EnablePort
  To Workspace1 : ToWorkspace  VariableName=EERAM_Current_Map_Backward  SaveFormat=Structure With Time  SampleTime=-1
      settings: Save2DSignal=2-D array (concatenate along first dimension)
  wires:
  In1/1 -> To Workspace1/1

== system APSA/APSA_OUTPUT/Subsystem2 ==
  In1 : Inport
  Enable : EnablePort
  To Workspace1 : ToWorkspace  VariableName=EERAM_Current_Map_Forward  SaveFormat=Structure With Time  SampleTime=-1
      settings: Save2DSignal=2-D array (concatenate along first dimension)
  wires:
  In1/1 -> To Workspace1/1
